simulink model "modelo_pacejka"  (R2025a)
settings: Solver=VariableStepAuto  StartTime=0.0  StopTime=10.0  RelTol=1e-3
undefined symbols (not defined in the file): a, b, delta_input, Fz_f_static, Fz_r_static, Iz, m, vx
settings Model: Creator=Anderson  LastModifiedBy=Anderson

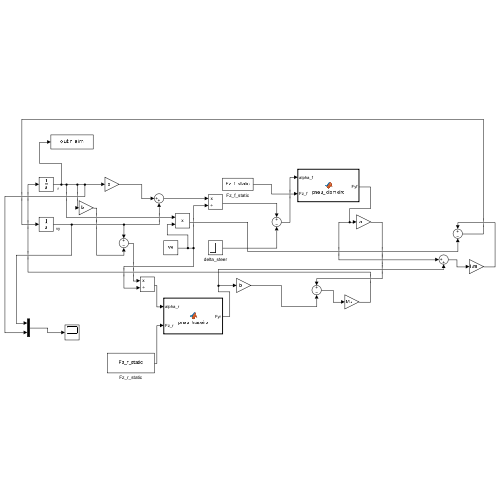
[thumbnail: Simulink's stored preview of the top-level diagram]
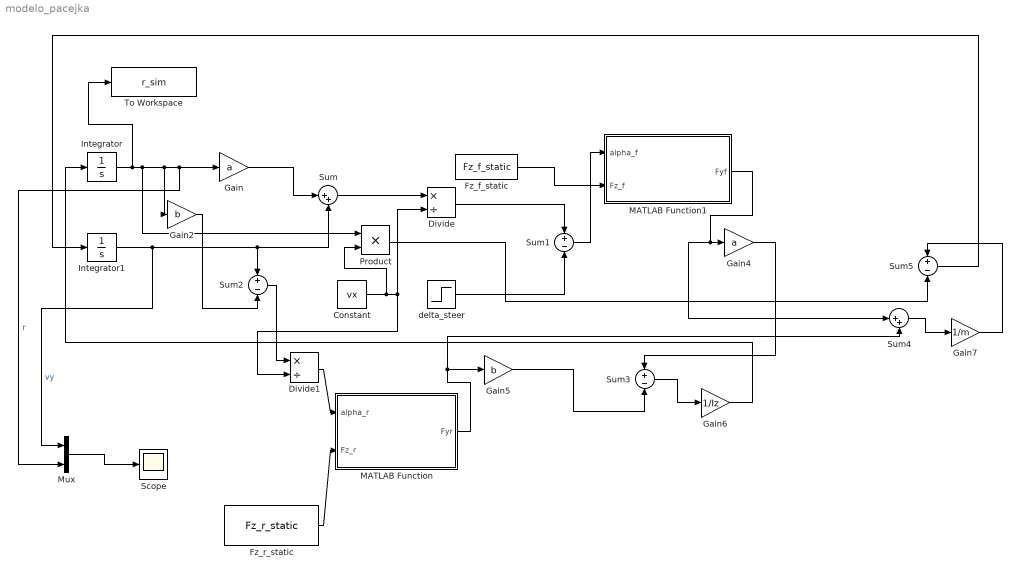
== system modelo_pacejka ==
  Constant : Constant  Value=vx
  Divide : Product  Inputs=*/
  Divide1 : Product  Inputs=*/
  Fz_f_static : Constant  Value=Fz_f_static
  Fz_r_static : Constant  Value=Fz_r_static
  Gain : Gain  Gain=a
  Gain2 : Gain  Gain=b
  Gain4 : Gain  Gain=a
  Gain5 : Gain  Gain=b
  Gain6 : Gain  Gain=1/Iz
  Gain7 : Gain  Gain=1/m
  Integrator : Integrator
  Integrator1 : Integrator
  MATLAB Function : MATLAB Function  TreatAsAtomicUnit=on
  MATLAB Function1 : MATLAB Function  TreatAsAtomicUnit=on
  Mux : Mux  Inputs=2
  Product : Product
  Scope : Scope
  Sum : Sum  Inputs=|++
  Sum{1..3,5} (4 alike) : Sum  Inputs=+-
  Sum4 : Sum  Inputs=|++
  To Workspace : ToWorkspace  VariableName=r_sim  SaveFormat=Timeseries  SampleTime=-1
  delta_steer : Step  After=delta_input  SampleTime=0
  wires:
  Integrator/1 -> To Workspace/1, Product/1, Gain2/1, Mux/2, Gain/1  "r"
  Integrator1/1 -> Mux/1, Sum2/1, Sum/2  "vy"
  Gain/1 -> Sum/1
  Sum/1 -> Divide/1
  Constant/1 -> Product/2, Divide1/2, Divide/2
  Divide/1 -> Sum1/1
  delta_steer/1 -> Sum1/2
  Sum1/1 -> MATLAB Function1/1(alpha_f)
  Gain2/1 -> Sum2/2
  MATLAB Function1/1(Fyf) -> Sum4/1, Gain4/1
  MATLAB Function/1(Fyr) -> Sum4/2, Gain5/1
  Gain4/1 -> Sum3/1
  Gain5/1 -> Sum3/2
  Sum3/1 -> Gain6/1
  Gain6/1 -> Integrator/1
  Sum4/1 -> Gain7/1
  Gain7/1 -> Sum5/1
  Product/1 -> Sum5/2
  Sum5/1 -> Integrator1/1
  Mux/1 -> Scope/1
  Sum2/1 -> Divide1/1
  Divide1/1 -> MATLAB Function/1(alpha_r)
  Fz_f_static/1 -> MATLAB Function1/2(Fz_f)
  Fz_r_static/1 -> MATLAB Function/2(Fz_r)

== matlab function modelo_pacejka/MATLAB Function ==
  data: alpha_r input; Fyr output; Fz_r input
function Fyr = pneu_traseiro(alpha_r, Fz_r)
% CÓDIGO CORRIGIDO E AUTOSSUFICIENTE
% Calcula a Força Lateral usando a Magic Formula de Pacejka.

% Coeficientes de Pacejka definidos diretamente aqui dentro
B = 10;
C = 1.9;
D_mult = 1.0; % Multiplicador do Pico de Aderência
E = 0.97;

% O pico da aderência (D) depende da carga vertical (Fz)
D = D_mult * Fz_r;

% Magic Formula de Pacejka (usando radianos)
phi = (1 - E) * alpha_r + (E / B) * atan(B * alpha_r);
Fyr_mag = D * sin(C * atan(B * phi));

% A força lateral é oposta ao ângulo de deriva
Fyr = -Fyr_mag;

end

== matlab function modelo_pacejka/MATLAB Function1 ==
  data: alpha_f input; Fyf output; Fz_f input
function Fyf = pneu_dianteiro(alpha_f, Fz_f)
% CÓDIGO CORRIGIDO E AUTOSSUFICIENTE
% Calcula a Força Lateral usando a Magic Formula de Pacejka.

% Coeficientes de Pacejka definidos diretamente aqui dentro
B = 10;
C = 1.9;
D_mult = 1.0; % Multiplicador do Pico de Aderência
E = 0.97;

% O pico da aderência (D) depende da carga vertical (Fz)
D = D_mult * Fz_f;

% Magic Formula de Pacejka (usando radianos)
phi = (1 - E) * alpha_f + (E / B) * atan(B * alpha_f);
Fyf_mag = D * sin(C * atan(B * phi));

% A força lateral é oposta ao ângulo de deriva
Fyf = -Fyf_mag;

end
